simulink model "XY_Inertial_To_XY_Body"  (R2019b)
settings: Solver=FixedStepAuto  StartTime=0.0  StopTime=200  FixedStep=0.001  RelTol=1e-3
PreLoadFcn:
  | cd D:\Aerospace\Model_Based_Design\Version_2.0
  | 
  | % This function reads the quad's parameters from the excel sheet.
  | 
  | data = xlsread('Tarek Deif''s Quad','B2:B9');
  | 
  | Quad.m = data(1);
  | Ixx =    data(2);
  | Iyy =    data(3);
  | Izz =    data(4);
  | g =      data(5);
  | Quad.b = data(6);
  | Quad.d = data(7);
  | Quad.h = data(8);
  | 
  | Quad.I = [Ixx,   0,   0;...
  |             0, Iyy,   0;...
  |             0,   0, Izz];
  | 
  | Quad.Omega_nom = sqrt(Quad.m*g/4/Quad.b);
  | 
  | Quad.mixer = [   0,  0.5, -0.25, 0.25;...
  |               -0.5,    0,  0.25, 0.25;...
  |                  0, -0.5, -0.25, 0.25;...
  |                0.5,    0,  0.25, 0.25];
settings Model: Creator=Mahmoud A. Moustafa  LastModifiedBy=Mahmoud A. Moustafa
settings DataIOCC: SaveOutput=off  SaveTime=off

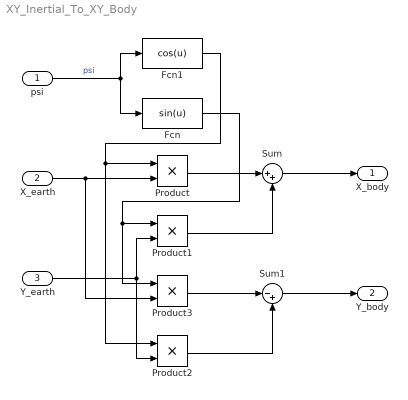
== system XY_Inertial_To_XY_Body ==
  psi : Inport  OutDataTypeStr=double  PortDimensions=[1 1]  SampleTime=0
  X_earth : Inport  Port=2  OutDataTypeStr=double  PortDimensions=1  SampleTime=0
  Y_earth : Inport  Port=3  OutDataTypeStr=double  PortDimensions=1  SampleTime=0
  Fcn : Fcn  Expr=sin(u)
  Fcn1 : Fcn  Expr=cos(u)
  Product{,1..3} (4 alike) : Product
  Sum : Sum  Inputs=|++
  Sum1 : Sum  Inputs=|-+
  X_body : Outport  OutDataTypeStr=double  PortDimensions=[1 1]  SampleTime=0
  Y_body : Outport  Port=2  OutDataTypeStr=double  PortDimensions=[1 1]  SampleTime=0
  wires:
  psi/1 -> Fcn/1, Fcn1/1  "psi"
  Product2/1 -> Sum1/2
  Y_earth/1 -> Product2/2, Product1/2
  X_earth/1 -> Product3/2, Product/2
  Fcn1/1 -> Product2/1, Product/1
  Fcn/1 -> Product3/1, Product1/1
  Product/1 -> Sum/1
  Product1/1 -> Sum/2
  Product3/1 -> Sum1/1
  Sum/1 -> X_body/1
  Sum1/1 -> Y_body/1
